simulink model "ysw15_3"  (R2014a)
settings: Solver=ode45  StartTime=0.0  StopTime=10.0  RelTol=1e-3
values from neighbouring files (symbols this model uses):
  A = [0,1,0,-1 ... (first row only)    [ysw15_4.m]    (also in ysw15_5.m)
  B = [0,0,1,0]'    [ysw15_4.m]    (also in ysw15_5.m)
  C = [-8.3859,-4.0703,7.6711,0.1549 ... (first row only)    [ysw15_4.m]    (also in ysw15_5.m = [-66.667,-4.083,0,4.083)
  D = [0,0,0]'    [ysw15_4.m]    (also in ysw15_5.m)
libraries: simulink x1
settings Model: Creator=ii  LastModifiedBy=ii
settings SolverCC: ZeroCrossAlgorithm=Adaptive
settings DebuggingCC: UnderspecifiedInitializationDetection=Classic

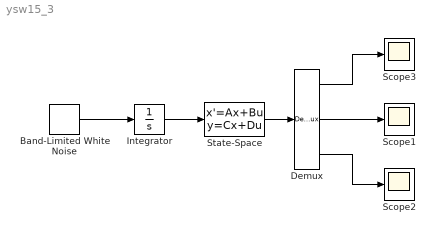
== system ysw15_3 ==
  Band-Limited White Noise : simulink/Sources/Band-Limited White Noise  Cov=[0.1]  Ts=0.1  seed=[23341]
  Demux : Demux  Outputs=3
  Integrator : Integrator
  Scope1 : Scope
  Scope2 : Scope
  Scope3 : Scope
      settings: SaveName=ScopeData3
  State-Space : StateSpace  A=A  B=B  C=C  D=D  X0=0
  wires:
  State-Space/1 -> Demux/1
  Demux/1 -> Scope3/1
  Demux/2 -> Scope1/1
  Demux/3 -> Scope2/1
  Integrator/1 -> State-Space/1
  Band-Limited White Noise/1 -> Integrator/1
